simulink model "ssc_battery_management_R2020a"  (R2020a)
settings: Solver=daessc  StartTime=0.0  StopTime=2000  FixedStep=0.1  MinStep=1e-6  RelTol=1e-5  EnableMultiTasking=on
PreLoadFcn:
  | ModelPath = fileparts(get_param(bdroot,'FileName'));
  | addpath(ModelPath);
  | 
  | ssc_battery_management_R2012b_ini
values from neighbouring files (symbols this model uses):
  AltData100AMaxCurrent =     [AlternatorTableData.mat]
  AltData100AVoltage =     [AlternatorTableData.mat]
  AltData80AMaxCurrent =     [AlternatorTableData.mat]
  AltData80AVoltage =     [AlternatorTableData.mat]
  Kt = [0.80,1.10,1.20,1.12;]    [ssc_lead_acid_battery_50Ah_ini.m]    (also in ssc_lead_acid_battery_80Ah_ini.m)
  Kt_Temps = [25 40 60 75]    [ssc_lead_acid_battery_50Ah_ini.m]    (also in ssc_lead_acid_battery_80Ah_ini.m)
  theta_f = -40    [ssc_lead_acid_battery_50Ah_ini.m]    (also in ssc_lead_acid_battery_80Ah_ini.m)
  theta_init = 25    [ssc_lead_acid_battery_50Ah_ini.m]    (also in ssc_lead_acid_battery_80Ah_ini.m)
undefined symbols (not defined in the file or in its folder): beta, center, DiscIntNeverNeededParam, exponent, polyTerms, sigbuilder_block, WendlandNumTerms, width
libraries: fl_lib x130, LeadAcidBattery_lib x36, nesl_utility x28, simulink x6
(part 1 of 4)
settings Model: Creator=smiller  LastModifiedBy=rjack
settings SolverCC: MaxConsecutiveMinStep=10  ZeroCrossAlgorithm=Adaptive  SolverResetMethod=Robust
settings DataIOCC: LimitDataPoints=on  SaveFormat=Array  SignalLoggingSaveFormat=ModelDataLogs  SignalLoggingName=sigsOut
settings OptimizationCC: ExpressionDepthLimit=2147483647  InitFltsAndDblsToZero=on  LifeSpan=inf
settings DebuggingCC: AlgebraicLoopMsg=none  SaveWithParameterizedLinksMsg=none  SignalResolutionControl=TryResolveAllWithWarning  IgnoredZcDiagnostic=none  MultiTaskDSMMsg=warning  MultiTaskCondExecSysMsg=none  StateNameClashWarn=warning  SFUnexpectedBacktrackingDiag=warning  SFNoUnconditionalDefaultTransitionDiag=warning  SFExecutionAtInitializationDiag=none  ArithmeticOperatorsInVariantConditions=warning
settings HardwareCC: ProdBitPerPointer=32  ProdBitPerSizeT=32  ProdBitPerPtrDiffT=32  ProdLargestAtomicFloat=None  ProdIntDivRoundTo=Undefined  ProdEndianess=Unspecified  ProdWordSize=32  ProdHWDeviceType=32-bit Generic  TargetBitPerPointer=64  TargetBitPerSizeT=64  TargetBitPerPtrDiffT=64  TargetLongLongMode=on  TargetIntDivRoundTo=Zero  TargetEndianess=LittleEndian  TargetWordSize=64  TargetHWDeviceType=MATLAB Host  ProdEqTarget=off
settings ModelReferenceCC: PropagateSignalLabelsOutOfModel=off
settings SFSimCC: SimUseLocalCustomCode=off  SimParseCustomCode=off  CustomCodeUndefinedFunction=UseInterfaceOnly
settings RTWCC: RTWUseLocalCustomCode=off
settings CodeAppCC: StateflowObjectComments=on
settings GRTTargetCC: TargetFcnLib=ansi_tfl_tmw.mat  TargetLangStandard=C89/C90 (ANSI)  CombineOutputUpdateFcns=off  GRTInterface=on
settings ConfigComp: CovMetricSettings=dw  CovHtmlReporting=on  CovSaveCumulativeToWorkspaceVar=on  CovSaveSingleToWorkspaceVar=on  CovExternalEMLEnable=off
settings SimscapeCC: SimscapeNormalizeSystem=off

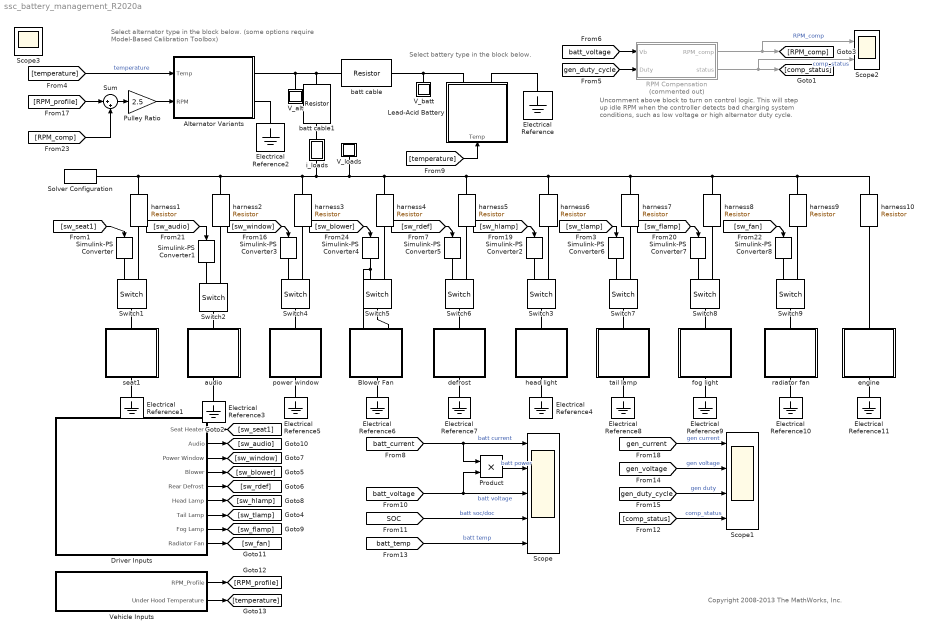
== system ssc_battery_management_R2020a ==
  note: Uncomment above block to turn on control logic.
      | This will step up idle RPM when the controller
      | detects bad charging system conditions, such
      | as low voltage or high alternator duty cycle.
  note: Copyright 2008-2013 The MathWorks, Inc.
  note: Select alternator type in the block below.
      | (some options require Model-Based Calibration Toolbox)
  note: Select battery type in the block below.
  Alternator Variants : Subsystem  Variant=on  mask(Alternator Variants){alt_type=80A (Lookup Tables), i_init=30}
      mask prompts: alt_type "Alternator Size and Type"; i_init "Initial Current (Amperes)"
      mask help:
      | Select from different alternator sizes and types. The Alternator Type selection will update the variable AlternatorSelection in the base workspace, which triggers the variant selection. Look under the mask to view the different alternator models. The initial current sets the initial condition of the alternator's output.
      |
      | The MBC alternator selections require Model-Based Calibration Toolbox to be installed.
      mask init:
      | assignin('base','AlternatorSelection',alt_type)
      mask TypeOptions alt_type: 80A (Lookup Tables) | 100A (Lookup Tables) | 80A (MBC Toolbox - high fidelity) | 100A (MBC Toolbox - high fidelity)
  Blower Fan : Subsystem  mask{steps=[1 2 3 4], current=[2.6 5.8 10 15.1; 2.5 6.4 10.9 16.4; 3.2 7.2 12.3 18.5], voltage=[11 12 13.5]}
      mask Display:
      | plot([45.5890141893179;79.6036154497415;90.9418158698828;113.618216710165;136.294617550448;158.97101839073;181.647419231013;204.323820071295;227.000220911577;249.67662175186;261.014822172001;295.029423432425], [85.2727156598121;85.2727156598121;107.949116500095;62.5963148195297;107.949116500095;62.5963148195297;107.949116500095;62.5963148195297;107.949116500095;62.5963148195297;85.2727156598121;85.2727156598121])
      | plot([0.236212508752999;45.5890141893179;45.5890141893179], [56.927214609459;56.927214609459;85.2727156598121])
      | plot([295.029423432425;295.029423432425;340.38222511299], [85.2727156598121;113.618216710165;113.618216710165])
      | plot([0.236212508752999;45.5890141893179;102.280016290024;124.956417130306;232.669321121648], [170.309218810871;170.309218810871;170.309218810871;141.963717760518;20.0780632440001])
      | plot([209.992920281366;232.669321121648;232.669321121648], [20.0780632440001;20.0780632440001;42.7544640842825])
      | patch([5.6843418860808e-14;340.618437621743;340.618437621743;0;5.6843418860808e-14;0.472425017505941;0.472425017505941;340.146012604237;340.146012604237;0.472425017505941;5.6843418860808e-14], [227.23643342033;227.23643342033;0;0;227.23643342033;226.764008402824;0.472425017505884;0.472425017505884;226.764008402824;226.764008402824;227.23643342033], [1;1;1])
      | ;
      | color('red');
      | port_label('LConn', 1,'Step')
      | port_label('LConn', 2,'+')
      | port_label('RConn', 1,'-')
  Driver Inputs : Subsystem  Tag=STV Subsys  LoadFcn=sigbuilder_block('load');  StartFcn=sigbuilder_block('start');  StopFcn=sigbuilder_block('stop');  ClipboardFcn=sigbuilder_block('clipboard');  mask(Sigbuilder block){tuvar=[0:10]}
      mask help: Sigbuilder GUI
      mask init:
      | if ~strcmp(get_param(bdroot,'SimulationStatus'),'stopped') tuvar = sigbuilder_block('maskInit'); end
      settings: CopyFcn=sigbuilder_block('copy');  DeleteFcn=sigbuilder_block('delete');  ModelCloseFcn=sigbuilder_block('modelClose');  PreSaveFcn=sigbuilder_block('preSave');  PauseFcn=sigbuilder_block('pause')  ContinueFcn=sigbuilder_block('continue')  NameChangeFcn=sigbuilder_block('namechange');  OpenFcn=sigbuilder_block('open',[652.8 249 792.6 639 ]);  CloseFcn=sigbuilder_block('close');
      mask Display: plot(0, 0, 100, 100,[2, 2, 32, 32, 2], [68, 8, 8, 68, 68],[32, 2], [38, 38], [32, 19, 2],[53, 60, 44], [32, 17, 17, 2],[16, 16, 31, 31]);txt = getActiveGroup(gcbh);text(2, 100, txt,'verticalAlignment', 'top');
  Electrical Reference{,1..11} (12 alike) : fl_lib/Electrical/Electrical Elements/Electrical Reference
  Lead-Acid Battery : Subsystem  InitFcn=ssc_lead_acid_battery_50Ah_ini  mask(Lead-Acid Battery){battery_type=50}
      mask prompts: battery_type "Capacity (Ampere-hours)"
      mask help: Select from different battery sizes. The selection will run the corresponding parameter initialization file for the battery capacity selected.
      mask init:
      | switch battery_type
      |     case 1 %50 Ah
      |         ssc_lead_acid_battery_50Ah_ini;
      |     case 2 %80 Ah
      |         ssc_lead_acid_battery_80Ah_ini;
      | end
      mask TypeOptions battery_type: 50 | 80
      mask Display:
      | port_label('RConn',1,'+')
      | port_label('RConn',2,'-')
      | port_label('input',1,'Temp')
      | disp([battery_type ' Ah'])
  Product : Product  RndMeth=Zero
  Pulley Ratio : Gain  Gain=2.5
  RPM Compensation : Subsystem  Commented=on
  Scope : Scope  NumInputPorts=5
  Scope1 : Scope  NumInputPorts=4
  Scope2 : Scope  NumInputPorts=2
  Simulink-PS Converter{,1..8} (9 alike) : nesl_utility/Simulink-PS Converter  PhysicalDomain=network_engine_domain  SubClassName=ps_input  LeftPortType=input  RightPortType=output  PseudoPeriodic=off  Frequencies=[]  NoiseDistribution=none  NoiseParameters=[]  Unit=1  AffineConversion=off  FilteringAndDerivatives=zero  SimscapeFilterOrder=1  InputFilterTimeConstant=.001  UdotUserProvided=0
  Solver Configuration : nesl_utility/Solver Configuration  PhysicalDomain=network_engine_domain  SubClassName=solver  LeftPortType=input  RightPortType=generic  Tones=[]  Harmonics=[]  SimulateNoise=off  Profile=off  UseLocalSampling=off  EnableSwitchedLinearOptims=on  FrequencyDomain=off  UseCCode=off  RelTol=0.001  AbsTol=1e-06  MinStep=1e-09  ToWorkspace=off  RevertToSquareIcSolve=off  NumHomotopyIterations=100  PhasorMode=off  PhasorModeNumHarmonics=1  DoDC=off  ResidualTolerance=1e-6  UseLocalSolver=off  LocalSolverChoice=NE_BACKWARD_EULER_ADVANCER  LocalSolverSampleTime=.001  DoFixedCost=off  MaxNonlinIter=12  MaxModeIter=2  LinearAlgebra=Sparse  EquationFormulation=NE_TIME_EF  DelaysMemoryBudget=1024  AutomaticFiltering=on  FilteringTimeConstant=0.001  PartitionStorageMethod=AS_NEEDED  PartitionMemoryBudget=1024  PartitionMethod=FAST
  Sum : Sum  Inputs=|++
  Switch{1..9} (9 alike) : fl_lib/Electrical/Electrical Elements/Switch  R_closed=0.01 Ohm  G_open=1e-08 1/Ohm  Threshold=0  i_specify=off  i_priority=None  i=0 A  i_nominal_specify=off  i_nominal_unit=A  i_nominal_value=1  v_specify=off  v_priority=None  v=0 V  v_nominal_specify=off  v_nominal_unit=V  v_nominal_value=1
  V_alt : Subsystem  InitFcn=|
      | unit=get_param([gcb '/PS-S'],'Unit');
      | set_param(gcb, 'AttributesFormatString', strcat('[', unit,']'));
      mask help: Simscape Probe
      settings: AttributesFormatString=[V]
      settings: CopyFcn=|
      | set_param(gcb,'LinkStatus','inactive')
      | set_param(gcb,'LinkStatus','none')
      | set_param([gcb '/Goto'],'GotoTag', [get(gcbh,'name')])
      | 
      | set_param([gcb '/From'],'GotoTag', [get(gcbh,'name')])
      settings: NameChangeFcn=|
      | set_param([gcb '/Goto'],'GotoTag', [get(gcbh,'name')])
      | 
      | set_param([gcb '/From'],'GotoTag', [get(gcbh,'name')])
      settings: OpenFcn=|
      | open_system([gcb '/voltage']);
      | close_system(gcb);                    hh=findobj(allchild(0),'name','voltage');
      | ha=findobj(hh(1),'type','axes');
      | set(get(ha,'title'),'string',get(gcbh,'name'));
      | clear hh ha;
      mask Display: port_label('LConn', 1,'V');
  V_batt : Subsystem  InitFcn=|
      | unit=get_param([gcb '/PS-S'],'Unit');
      | set_param(gcb, 'AttributesFormatString', strcat('[', unit,']'));
      mask help: Simscape Probe
      settings: AttributesFormatString=[V]
      settings: CopyFcn=|
      | set_param(gcb,'LinkStatus','inactive')
      | set_param(gcb,'LinkStatus','none')
      | set_param([gcb '/Goto'],'GotoTag', [get(gcbh,'name')])
      | 
      | set_param([gcb '/From'],'GotoTag', [get(gcbh,'name')])
      settings: NameChangeFcn=|
      | set_param([gcb '/Goto'],'GotoTag', [get(gcbh,'name')])
      | 
      | set_param([gcb '/From'],'GotoTag', [get(gcbh,'name')])
      settings: OpenFcn=|
      | open_system([gcb '/voltage']);
      | close_system(gcb);                    hh=findobj(allchild(0),'name','voltage');
      | ha=findobj(hh(1),'type','axes');
      | set(get(ha,'title'),'string',get(gcbh,'name'));
      | clear hh ha;
      mask Display: port_label('LConn', 1,'V');
  V_loads : Subsystem  InitFcn=|
      | unit=get_param([gcb '/PS-S'],'Unit');
      | set_param(gcb, 'AttributesFormatString', strcat('[', unit,']'));
      mask help: Simscape Probe
      settings: AttributesFormatString=[V]
      settings: CopyFcn=|
      | set_param(gcb,'LinkStatus','inactive')
      | set_param(gcb,'LinkStatus','none')
      | set_param([gcb '/Goto'],'GotoTag', [get(gcbh,'name')])
      | 
      | set_param([gcb '/From'],'GotoTag', [get(gcbh,'name')])
      settings: NameChangeFcn=|
      | set_param([gcb '/Goto'],'GotoTag', [get(gcbh,'name')])
      | 
      | set_param([gcb '/From'],'GotoTag', [get(gcbh,'name')])
      settings: OpenFcn=|
      | open_system([gcb '/voltage']);
      | close_system(gcb);                    hh=findobj(allchild(0),'name','voltage');
      | ha=findobj(hh(1),'type','axes');
      | set(get(ha,'title'),'string',get(gcbh,'name'));
      | clear hh ha;
      mask Display: port_label('LConn', 1,'V');
  Vehicle Inputs : Subsystem  Tag=STV Subsys  LoadFcn=sigbuilder_block('load');  StartFcn=sigbuilder_block('start');  StopFcn=sigbuilder_block('stop');  ClipboardFcn=sigbuilder_block('clipboard');  mask(Sigbuilder block){tuvar=[0:10]}
      mask help: Sigbuilder GUI
      mask init:
      | if ~strcmp(get_param(bdroot(gcbh),'SimulationStatus'),'stopped') tuvar = sigbuilder_block('maskInit'); end
      settings: CopyFcn=sigbuilder_block('copy');  DeleteFcn=sigbuilder_block('delete');  ModelCloseFcn=sigbuilder_block('modelClose');  PreSaveFcn=sigbuilder_block('preSave');  PauseFcn=sigbuilder_block('pause')  ContinueFcn=sigbuilder_block('continue')  NameChangeFcn=sigbuilder_block('namechange');  OpenFcn=sigbuilder_block('open',[910.5 430.5 511.5 350.25 ]);  CloseFcn=sigbuilder_block('close');
      mask Display: plot(0, 0, 100, 100,[2, 2, 32, 32, 2], [68, 8, 8, 68, 68],[32, 2], [38, 38], [32, 19, 2],[53, 60, 44], [32, 17, 17, 2],[16, 16, 31, 31]);txt = getActiveGroup(gcbh);text(2, 100, txt,'verticalAlignment', 'top');
  audio : Subsystem  mask{current=[7.64 8.33 9.38], voltage=[11 12 13.5]}
      mask Display:
      | plot([0.236212508752942;34.2508137691766;45.5890141893178;68.2654150296003;90.9418158698827;113.618216710165;136.294617550448;158.97101839073;181.647419231012;204.323820071295;215.662020491436;249.67662175186], [85.2727156598121;85.2727156598121;107.949116500095;62.5963148195297;107.949116500095;62.5963148195297;107.949116500095;62.5963148195297;107.949116500095;62.5963148195297;85.2727156598121;85.2727156598121])
      | plot([50;200], [155;20])
      | plot([170;200;200], [25;20;45])
      | patch([0;249.912834260613;249.912834260613;0;0;0.472425017505884;0.472425017505884;249.440409243107;249.440409243107;0.472425017505884;0], [170.545431319624;170.545431319624;0;0;170.545431319624;170.073006302118;0.472425017505884;0.472425017505884;170.073006302118;170.073006302118;170.545431319624], [1;1;1])
      | ;
      | color('red');
      | port_label('LConn', 1,'+')
      | port_label('RConn', 1,'-')
  batt cable1 : fl_lib/Electrical/Electrical Elements/Resistor  R=0.003 Ohm  i_specify=off  i_priority=None  i=0 A  i_nominal_specify=off  i_nominal_unit=A  i_nominal_value=1  v_specify=off  v_priority=None  v=0 V  v_nominal_specify=off  v_nominal_unit=V  v_nominal_value=1
  batt cable : fl_lib/Electrical/Electrical Elements/Resistor  R=0.03 Ohm  i_specify=off  i_priority=None  i=0 A  i_nominal_specify=off  i_nominal_unit=A  i_nominal_value=1  v_specify=off  v_priority=None  v=0 V  v_nominal_specify=off  v_nominal_unit=V  v_nominal_value=1
  defrost : Subsystem  mask{current=[22.92 25 28.13], voltage=[11 12 13.5]}
      mask Display:
      | plot([0.236212508752942;34.2508137691766;45.5890141893178;68.2654150296003;90.9418158698827;113.618216710165;136.294617550448;158.97101839073;181.647419231012;204.323820071295;215.662020491436;249.67662175186], [85.2727156598121;85.2727156598121;107.949116500095;62.5963148195297;107.949116500095;62.5963148195297;107.949116500095;62.5963148195297;107.949116500095;62.5963148195297;85.2727156598121;85.2727156598121])
      | plot([50;200], [155;20])
      | plot([170;200;200], [25;20;45])
      | patch([0;249.912834260613;249.912834260613;0;0;0.472425017505884;0.472425017505884;249.440409243107;249.440409243107;0.472425017505884;0], [170.545431319624;170.545431319624;0;0;170.545431319624;170.073006302118;0.472425017505884;0.472425017505884;170.073006302118;170.073006302118;170.545431319624], [1;1;1])
      | ;
      | color('red');
      | port_label('LConn', 1,'+')
      | port_label('RConn', 1,'-')
  engine : Subsystem  mask{current=[11.8 12.9 14.5], voltage=[11 12 13.5]}
      mask Display:
      | plot([0.236212508752942;34.2508137691766;45.5890141893178;68.2654150296003;90.9418158698827;113.618216710165;136.294617550448;158.97101839073;181.647419231012;204.323820071295;215.662020491436;249.67662175186], [85.2727156598121;85.2727156598121;107.949116500095;62.5963148195297;107.949116500095;62.5963148195297;107.949116500095;62.5963148195297;107.949116500095;62.5963148195297;85.2727156598121;85.2727156598121])
      | plot([50;200], [155;20])
      | plot([170;200;200], [25;20;45])
      | patch([0;249.912834260613;249.912834260613;0;0;0.472425017505884;0.472425017505884;249.440409243107;249.440409243107;0.472425017505884;0], [170.545431319624;170.545431319624;0;0;170.545431319624;170.073006302118;0.472425017505884;0.472425017505884;170.073006302118;170.073006302118;170.545431319624], [1;1;1])
      | ;
      | color('red');
      | port_label('LConn', 1,'+')
      | port_label('RConn', 1,'-')
  fog light : Subsystem  mask{current=[7.64 8.33 9.38], voltage=[11 12 13.5]}
      mask Display:
      | plot([0.236212508752942;34.2508137691766;45.5890141893178;68.2654150296003;90.9418158698827;113.618216710165;136.294617550448;158.97101839073;181.647419231012;204.323820071295;215.662020491436;249.67662175186], [85.2727156598121;85.2727156598121;107.949116500095;62.5963148195297;107.949116500095;62.5963148195297;107.949116500095;62.5963148195297;107.949116500095;62.5963148195297;85.2727156598121;85.2727156598121])
      | plot([50;200], [155;20])
      | plot([170;200;200], [25;20;45])
      | patch([0;249.912834260613;249.912834260613;0;0;0.472425017505884;0.472425017505884;249.440409243107;249.440409243107;0.472425017505884;0], [170.545431319624;170.545431319624;0;0;170.545431319624;170.073006302118;0.472425017505884;0.472425017505884;170.073006302118;170.073006302118;170.545431319624], [1;1;1])
      | ;
      | color('red');
      | port_label('LConn', 1,'+')
      | port_label('RConn', 1,'-')
  harness{1..8,10} (9 alike) : fl_lib/Electrical/Electrical Elements/Resistor  R=0.05 Ohm  i_specify=off  i_priority=None  i=0 A  i_nominal_specify=off  i_nominal_unit=A  i_nominal_value=1  v_specify=off  v_priority=None  v=0 V  v_nominal_specify=off  v_nominal_unit=V  v_nominal_value=1
  harness9 : fl_lib/Electrical/Electrical Elements/Resistor  R=0.01 Ohm  i_specify=off  i_priority=None  i=0 A  i_nominal_specify=off  i_nominal_unit=A  i_nominal_value=1  v_specify=off  v_priority=None  v=0 V  v_nominal_specify=off  v_nominal_unit=V  v_nominal_value=1
  head light : Subsystem  mask{current=[7.64 8.33 9.38], voltage=[11 12 13.5]}
      mask Display:
      | plot([0.236212508752942;34.2508137691766;45.5890141893178;68.2654150296003;90.9418158698827;113.618216710165;136.294617550448;158.97101839073;181.647419231012;204.323820071295;215.662020491436;249.67662175186], [85.2727156598121;85.2727156598121;107.949116500095;62.5963148195297;107.949116500095;62.5963148195297;107.949116500095;62.5963148195297;107.949116500095;62.5963148195297;85.2727156598121;85.2727156598121])
      | plot([50;200], [155;20])
      | plot([170;200;200], [25;20;45])
      | patch([0;249.912834260613;249.912834260613;0;0;0.472425017505884;0.472425017505884;249.440409243107;249.440409243107;0.472425017505884;0], [170.545431319624;170.545431319624;0;0;170.545431319624;170.073006302118;0.472425017505884;0.472425017505884;170.073006302118;170.073006302118;170.545431319624], [1;1;1])
      | ;
      | color('red');
      | port_label('LConn', 1,'+')
      | port_label('RConn', 1,'-')
  i_loads : Subsystem  InitFcn=|
      | unit=get_param([gcb '/PS-S'],'Unit');
      | set_param(gcb, 'AttributesFormatString', strcat('[', unit,']'));
      mask help: Simscape Probe
      settings: AttributesFormatString=[A]
      settings: CopyFcn=|
      | set_param(gcb,'LinkStatus','inactive')
      | set_param(gcb,'LinkStatus','none')
      | set_param([gcb '/Goto'],'GotoTag', [get(gcbh,'name')])
      | 
      | set_param([gcb '/From'],'GotoTag', [get(gcbh,'name')])
      settings: NameChangeFcn=|
      | set_param([gcb '/Goto'],'GotoTag', [get(gcbh,'name')])
      | 
      | set_param([gcb '/From'],'GotoTag', [get(gcbh,'name')])
      settings: OpenFcn=|
      | open_system([gcb '/current']);
      | close_system(gcb);                    hh=findobj(allchild(0),'name','current');
      | ha=findobj(hh(1),'type','axes');
      | set(get(ha,'title'),'string',get(gcbh,'name'));
      | clear hh ha;
      mask Display:
      | patch([0.5 1 0.5], [0.25 .5 0.75],[0 0 0])
      | plot([0,0.5],[0.5,0.5]);
  power window : Subsystem  mask{current=[7.64 8.33 9.38], voltage=[11 12 13.5]}
      mask Display:
      | plot([0.236212508752942;34.2508137691766;45.5890141893178;68.2654150296003;90.9418158698827;113.618216710165;136.294617550448;158.97101839073;181.647419231012;204.323820071295;215.662020491436;249.67662175186], [85.2727156598121;85.2727156598121;107.949116500095;62.5963148195297;107.949116500095;62.5963148195297;107.949116500095;62.5963148195297;107.949116500095;62.5963148195297;85.2727156598121;85.2727156598121])
      | plot([50;200], [155;20])
      | plot([170;200;200], [25;20;45])
      | patch([0;249.912834260613;249.912834260613;0;0;0.472425017505884;0.472425017505884;249.440409243107;249.440409243107;0.472425017505884;0], [170.545431319624;170.545431319624;0;0;170.545431319624;170.073006302118;0.472425017505884;0.472425017505884;170.073006302118;170.073006302118;170.545431319624], [1;1;1])
      | ;
      | color('red');
      | port_label('LConn', 1,'+')
      | port_label('RConn', 1,'-')
  radiator fan : Subsystem  mask{current=[15.28 16.67 18.75], voltage=[11 12 13.5]}
      mask Display:
      | plot([0.236212508752942;34.2508137691766;45.5890141893178;68.2654150296003;90.9418158698827;113.618216710165;136.294617550448;158.97101839073;181.647419231012;204.323820071295;215.662020491436;249.67662175186], [85.2727156598121;85.2727156598121;107.949116500095;62.5963148195297;107.949116500095;62.5963148195297;107.949116500095;62.5963148195297;107.949116500095;62.5963148195297;85.2727156598121;85.2727156598121])
      | plot([50;200], [155;20])
      | plot([170;200;200], [25;20;45])
      | patch([0;249.912834260613;249.912834260613;0;0;0.472425017505884;0.472425017505884;249.440409243107;249.440409243107;0.472425017505884;0], [170.545431319624;170.545431319624;0;0;170.545431319624;170.073006302118;0.472425017505884;0.472425017505884;170.073006302118;170.073006302118;170.545431319624], [1;1;1])
      | ;
      | color('red');
      | port_label('LConn', 1,'+')
      | port_label('RConn', 1,'-')
  seat1 : Subsystem  mask{current=[11.16 12.5 14.06], voltage=[11 12 13.5]}
      mask Display:
      | plot([0.236212508752942;34.2508137691766;45.5890141893178;68.2654150296003;90.9418158698827;113.618216710165;136.294617550448;158.97101839073;181.647419231012;204.323820071295;215.662020491436;249.67662175186], [85.2727156598121;85.2727156598121;107.949116500095;62.5963148195297;107.949116500095;62.5963148195297;107.949116500095;62.5963148195297;107.949116500095;62.5963148195297;85.2727156598121;85.2727156598121])
      | plot([50;200], [155;20])
      | plot([170;200;200], [25;20;45])
      | patch([0;249.912834260613;249.912834260613;0;0;0.472425017505884;0.472425017505884;249.440409243107;249.440409243107;0.472425017505884;0], [170.545431319624;170.545431319624;0;0;170.545431319624;170.073006302118;0.472425017505884;0.472425017505884;170.073006302118;170.073006302118;170.545431319624], [1;1;1])
      | ;
      | color('red');
      | port_label('LConn', 1,'+')
      | port_label('RConn', 1,'-')
  tail lamp : Subsystem  mask{current=[4.7 4.9 5.15], voltage=[11 12 13.5]}
      mask Display:
      | plot([0.236212508752942;34.2508137691766;45.5890141893178;68.2654150296003;90.9418158698827;113.618216710165;136.294617550448;158.97101839073;181.647419231012;204.323820071295;215.662020491436;249.67662175186], [85.2727156598121;85.2727156598121;107.949116500095;62.5963148195297;107.949116500095;62.5963148195297;107.949116500095;62.5963148195297;107.949116500095;62.5963148195297;85.2727156598121;85.2727156598121])
      | plot([50;200], [155;20])
      | plot([170;200;200], [25;20;45])
      | patch([0;249.912834260613;249.912834260613;0;0;0.472425017505884;0.472425017505884;249.440409243107;249.440409243107;0.472425017505884;0], [170.545431319624;170.545431319624;0;0;170.545431319624;170.073006302118;0.472425017505884;0.472425017505884;170.073006302118;170.073006302118;170.545431319624], [1;1;1])
      | ;
      | color('red');
      | port_label('LConn', 1,'+')
      | port_label('RConn', 1,'-')
  Scope3 : Scope
  wires:
  [batt_current] -> Scope/1, Product/1  "batt current"
  [batt_voltage] -> Scope/3, Product/2  "batt voltage"
  [batt_temp] -> Scope/5  "batt temp"
  Driver Inputs/5(Rear Defrost) -> [sw_rdef]
  Driver Inputs/3(Power Window) -> [sw_window]
  Driver Inputs/6(Head Lamp) -> [sw_hlamp]
  Driver Inputs/8(Fog Lamp) -> [sw_flamp]
  Driver Inputs/2(Audio) -> [sw_audio]
  Driver Inputs/1(Seat Heater) -> [sw_seat1]
  Driver Inputs/9(Radiator Fan) -> [sw_fan]
  [sw_seat1] -> Simulink-PS Converter/1
  [SOC] -> Scope/4  "batt soc/doc"
  Product/1 -> Scope/2  "batt power"
  Vehicle Inputs/1(RPM_Profile) -> [RPM_profile]
  Vehicle Inputs/2(Under Hood Temperature) -> [temperature]
  [temperature] -> Lead-Acid Battery/1(Temp)
  [temperature] -> Alternator Variants/1(Temp)  "temperature"
  Pulley Ratio/1 -> Alternator Variants/2(RPM)
  [sw_audio] -> Simulink-PS Converter1/1
  [sw_window] -> Simulink-PS Converter3/1
  [sw_blower] -> Simulink-PS Converter4/1
  [sw_rdef] -> Simulink-PS Converter5/1
  [sw_tlamp] -> Simulink-PS Converter6/1
  [sw_flamp] -> Simulink-PS Converter7/1
  [sw_fan] -> Simulink-PS Converter8/1
  [sw_hlamp] -> Simulink-PS Converter2/1
  Driver Inputs/7(Tail Lamp) -> [sw_tlamp]
  Driver Inputs/4(Blower) -> [sw_blower]
  [gen_duty_cycle] -> RPM Compensation/2(Duty)
  [batt_voltage] -> RPM Compensation/1(Vb)
  RPM Compensation/2(status) -> [comp_status], Scope2/2  "comp_status"
  RPM Compensation/1(RPM_comp) -> [RPM_comp], Scope2/1  "RPM_comp"
  [RPM_profile] -> Sum/1
  [RPM_comp] -> Sum/2
  Sum/1 -> Pulley Ratio/1
  [gen_current] -> Scope1/1  "gen current"
  [gen_voltage] -> Scope1/2  "gen voltage"
  [gen_duty_cycle] -> Scope1/3  "gen duty"
  [comp_status] -> Scope1/4  "comp_status"
  connections:
  Lead-Acid Battery/RConn2 -- Electrical Reference/LConn1
  Lead-Acid Battery/RConn1 -- batt cable/LConn1 -- V_batt/LConn1
  i_loads/RConn1 -- V_loads/LConn1 -- harness10/LConn1 -- harness9/LConn1 -- harness8/LConn1 -- harness7/LConn1 -- harness6/LConn1 -- harness5/LConn1 -- harness4/LConn1 -- harness3/LConn1 -- harness1/LConn1 -- Solver Configuration/RConn1 -- harness2/LConn1
  Electrical Reference1/LConn1 -- seat1/RConn1
  Simulink-PS Converter/RConn1 -- Switch1/RConn1
  harness1/RConn1 -- Switch1/RConn2
  seat1/LConn1 -- Switch1/LConn1
  engine/LConn1 -- harness10/RConn1
  Electrical Reference11/LConn1 -- engine/RConn1
  batt cable/RConn1 -- Alternator Variants/RConn1 -- V_alt/LConn1 -- batt cable1/LConn1
  Alternator Variants/RConn2 -- Electrical Reference2/LConn1
  Switch2/LConn1 -- audio/LConn1
  Simulink-PS Converter1/RConn1 -- Switch2/RConn1
  Electrical Reference3/LConn1 -- audio/RConn1
  Electrical Reference4/LConn1 -- head light/RConn1
  Simulink-PS Converter2/RConn1 -- Switch3/RConn1
  Switch3/LConn1 -- head light/LConn1
  Electrical Reference5/LConn1 -- power window/RConn1
  Switch4/LConn1 -- power window/LConn1
  Simulink-PS Converter3/RConn1 -- Switch4/RConn1
  Switch5/LConn1 -- Blower Fan/LConn2
  Electrical Reference6/LConn1 -- Blower Fan/RConn1
  Simulink-PS Converter5/RConn1 -- Switch6/RConn1
  Switch6/LConn1 -- defrost/LConn1
  Electrical Reference7/LConn1 -- defrost/RConn1
  harness7/RConn1 -- Switch7/RConn2
  Simulink-PS Converter6/RConn1 -- Switch7/RConn1
  Electrical Reference8/LConn1 -- tail lamp/RConn1
  Switch7/LConn1 -- tail lamp/LConn1
  harness8/RConn1 -- Switch8/RConn2
  Electrical Reference9/LConn1 -- fog light/RConn1
  Switch8/LConn1 -- fog light/LConn1
  Simulink-PS Converter7/RConn1 -- Switch8/RConn1
  Simulink-PS Converter8/RConn1 -- Switch9/RConn1
  Switch9/LConn1 -- radiator fan/LConn1
  Electrical Reference10/LConn1 -- radiator fan/RConn1
  harness9/RConn1 -- Switch9/RConn2
  harness5/RConn1 -- Switch6/RConn2
  Switch4/RConn2 -- harness3/RConn1
  harness6/RConn1 -- Switch3/RConn2
  harness2/RConn1 -- Switch2/RConn2
  Blower Fan/LConn1 -- Simulink-PS Converter4/RConn1 -- Switch5/RConn1
  Switch5/RConn2 -- harness4/RConn1
  batt cable1/RConn1 -- i_loads/LConn1

== system ssc_battery_management_R2020a/Alternator Variants ==
  note: 1) Only subsystems can be added as variant choices at this level
      | 2) Blocks cannot be connected at this level as connectivity is
      | automatically determined at simulation, based on the active variant
  note: Alternator Blocks - Lookup Tables
  note: Alternator Blocks - MBC
  Temp : Inport
  RPM : Inport  Port=2
  Alternator_100A_LUT : Subsystem  VariantControl=Alternator_100A_LUT
  Alternator_100A_MBC : Subsystem  VariantControl=Alternator_100A_MBC
  Alternator_80A_LUT : Subsystem  VariantControl=Alternator_80A_LUT
  Alternator_80A_MBC : Subsystem  VariantControl=Alternator_80A_MBC
  + : PMIOPort  Side=Right
  - : PMIOPort  Port=2  Side=Right

== system ssc_battery_management_R2020a/Blower Fan ==
  PS Lookup Table (2D) : fl_lib/Physical Signals/Lookup Tables/PS Lookup Table (2D)  x1=[0 voltage]' V  x2=steps  f="[voltage(1)./current(1,:);  (voltage'*ones(size(steps)))./current] Ohm"  interp_method=simscape.enum.interpolation.linear  extrap_method=simscape.enum.extrapolation.nearest
      settings: SourceProductBaseCode=SS
  Variable Resistor : fl_lib/Electrical/Electrical Elements/Variable Resistor  Rmin=0.01 Ohm  i_specify=off  i_priority=None  i=0 A  i_nominal_specify=off  i_nominal_unit=A  i_nominal_value=1  v_specify=off  v_priority=None  v=0 V  v_nominal_specify=off  v_nominal_unit=V  v_nominal_value=1
  Voltage Sensor : fl_lib/Electrical/Electrical Sensors/Voltage Sensor
  Step : PMIOPort  Tag=PMCPort  Side=Left
  + : PMIOPort  Tag=PMCPort  Port=2  Side=Left
  - : PMIOPort  Tag=PMCPort  Port=3  Side=Right
  connections:
  Step/RConn1 -- PS Lookup Table (2D)/LConn2
  Voltage Sensor/RConn1 -- PS Lookup Table (2D)/LConn1
  +/RConn1 -- Variable Resistor/LConn2 -- Voltage Sensor/LConn1
  -/RConn1 -- Variable Resistor/RConn1 -- Voltage Sensor/RConn2
  Variable Resistor/LConn1 -- PS Lookup Table (2D)/RConn1

== system ssc_battery_management_R2020a/Driver Inputs ==
  Demux : Demux  Tag=STV Demux  Outputs=9
      settings: DisplayOption=none
  FromWs : FromWorkspace  Tag=STV FromWs  VariableName=tuvar  ZeroCross=off
      SigBuilderData=|
      | dataSet(1).timeRange = [0 2000]
      | dataSet(1).name = 'USA'
      | dataSet(2).timeRange = [0 2000]
      | dataSet(2).name = 'Asia'
      | dataSet(3).timeRange = [0 2000]
      | dataSet(3).name = 'Europe'
      | sbobj.Groups(1).Name = 'USA'
      | sbobj.Groups(1).Signals(1).Name = 'Seat Heater'
      | sbobj.Groups(1).Signals(1).XData = [0 60 60 886 886 2000]
      | sbobj.Groups(1).Signals(1).YData = [0 0 1 1 0 0]
      | sbobj.Groups(1).Signals(2).Name = 'Audio'
      | sbobj.Groups(1).Signals(2).XData = [0 116 116 2000]
      | sbobj.Groups(1).Signals(2).YData = [0 0 1 1]
      | sbobj.Groups(1).Signals(3).Name = 'Power Window'
      | sbobj.Groups(1).Signals(3).XData = [0 728 728 740 740 786 786 800 800 2000]
      | sbobj.Groups(1).Signals(3).YData = [0 0 1 1 0 0 1 1 0 0]
      | sbobj.Groups(1).Signals(4).Name = 'Blower'
      | sbobj.Groups(1).Signals(4).XData = [0 50 50 136 136 384 384 820 820 1082 1082 2000]
      | sbobj.Groups(1).Signals(4).YData = [0 0 4 4 3 3 2 2 1 1 2 2]
      | sbobj.Groups(1).Signals(5).Name = 'Rear Defrost'
      | sbobj.Groups(1).Signals(5).XData = [0 20 20 436 436 2000]
      | sbobj.Groups(1).Signals(5).YData = [0 0 1 1 0 0]
      | sbobj.Groups(1).Signals(6).Name = 'Head Lamp'
      | sbobj.Groups(1).Signals(6).XData = [0 200 200 2000]
      | sbobj.Groups(1).Signals(6).YData = [0 0 1 1]
      | sbobj.Groups(1).Signals(7).Name = 'Tail Lamp'
      | sbobj.Groups(1).Signals(7).XData = [0 200 200 2000]
      | sbobj.Groups(1).Signals(7).YData = [0 0 1 1]
      | sbobj.Groups(1).Signals(8).Name = 'Fog Lamp'
      | sbobj.Groups(1).Signals(8).XData = [0 400 400 2000]
      | sbobj.Groups(1).Signals(8).YData = [0 0 1 1]
      | sbobj.Groups(1).Signals(9).Name = 'Radiator Fan'
      | sbobj.Groups(1).Signals(9).XData = [0 814 814 1424 1424 2000]
      | sbobj.Groups(1).Signals(9).YData = [0 0 1 1 0 0]
      | sbobj.Groups(1).TimeRange = [0 2000]
      | sbobj.Groups(2).Name = 'Asia'
      | sbobj.Groups(2).Signals(1).Name = 'Seat Heater'
      | sbobj.Groups(2).Signals(1).XData = [0 60 886 2000]
      | sbobj.Groups(2).Signals(1).YData = [0 0 0 0]
      | sbobj.Groups(2).Signals(2).Name = 'Audio'
      | sbobj.Groups(2).Signals(2).XData = [0 116 116 2000]
      | sbobj.Groups(2).Signals(2).YData = [0 0 1 1]
      | sbobj.Groups(2).Signals(3).Name = 'Power Window'
      | sbobj.Groups(2).Signals(3).XData = [0 312 312 330 330 1762 1762 1774 1774 2000]
      | sbobj.Groups(2).Signals(3).YData = [0 0 1 1 0 0 1 1 0 0]
      | sbobj.Groups(2).Signals(4).Name = 'Blower'
      | sbobj.Groups(2).Signals(4).XData = [0 50 50 136 136 282 282 820 820 1082 1082 2000]
      | sbobj.Groups(2).Signals(4).YData = [0 0 4 4 3 3 -0.1 -0.1 1 1 0 0]
      | sbobj.Groups(2).Signals(5).Name = 'Rear Defrost'
      | sbobj.Groups(2).Signals(5).XData = [0 20 436 2000]
      | sbobj.Groups(2).Signals(5).YData = [0 0 0 0]
      | sbobj.Groups(2).Signals(6).Name = 'Head Lamp'
      | sbobj.Groups(2).Signals(6).XData = [0 200 2000]
      | sbobj.Groups(2).Signals(6).YData = [0 0 0]
      | sbobj.Groups(2).Signals(7).Name = 'Tail Lamp'
      | sbobj.Groups(2).Signals(7).XData = [0 200 2000]
      | sbobj.Groups(2).Signals(7).YData = [0 0 0]
      | sbobj.Groups(2).Signals(8).Name = 'Fog Lamp'
      | sbobj.Groups(2).Signals(8).XData = [0 400 2000]
      | sbobj.Groups(2).Signals(8).YData = [0 0 0]
      | sbobj.Groups(2).Signals(9).Name = 'Radiator Fan'
      | sbobj.Groups(2).Signals(9).XData = [0 810 810 1538 1538 2000]
      | sbobj.Groups(2).Signals(9).YData = [0 0 1 1 0 0]
      | sbobj.Groups(2).TimeRange = [0 2000]
      | sbobj.Groups(3).Name = 'Europe'
      | sbobj.Groups(3).Signals(1).Name = 'Seat Heater'
      | sbobj.Groups(3).Signals(1).XData = [0 164 164 2000]
      | sbobj.Groups(3).Signals(1).YData = [0 0 1 1]
      | sbobj.Groups(3).Signals(2).Name = 'Audio'
      | sbobj.Groups(3).Signals(2).XData = [0 116 116 2000]
      | sbobj.Groups(3).Signals(2).YData = [0 0 1 1]
      | sbobj.Groups(3).Signals(3).Name = 'Power Window'
      | sbobj.Groups(3).Signals(3).XData = [0 728 728 740 740 786 786 800 800 1046 1046 1060 1060 1118 1118 1140 1140 2000]
      | sbobj.Groups(3).Signals(3).YData = [0 0 1 1 0 0 1 1 0 0 1 1 0 0 1 1 0 0]
      | sbobj.Groups(3).Signals(4).Name = 'Blower'
      | sbobj.Groups(3).Signals(4).XData = [0 50 50 136 136 384 384 820 820 1082 1082 2000]
      | sbobj.Groups(3).Signals(4).YData = [0 0 4 4 3 3 2 2 3 3 2 2]
      | sbobj.Groups(3).Signals(5).Name = 'Rear Defrost'
      | sbobj.Groups(3).Signals(5).XData = [0 20 20 496 496 972 972 1660 1660 2000]
      | sbobj.Groups(3).Signals(5).YData = [0 0 1 1 0 0 1 1 0 0]
      | sbobj.Groups(3).Signals(6).Name = 'Head Lamp'
      | sbobj.Groups(3).Signals(6).XData = [0 20 20 2000]
      | sbobj.Groups(3).Signals(6).YData = [0 0 1 1]
      | sbobj.Groups(3).Signals(7).Name = 'Tail Lamp'
      | sbobj.Groups(3).Signals(7).XData = [0 18 720 2000]
      | sbobj.Groups(3).Signals(7).YData = [0 0 0 0]
      | sbobj.Groups(3).Signals(8).Name = 'Fog Lamp'
      | sbobj.Groups(3).Signals(8).XData = [0 400 2000]
      | sbobj.Groups(3).Signals(8).YData = [0 0 0]
      | sbobj.Groups(3).Signals(9).Name = 'Radiator Fan'
      | sbobj.Groups(3).Signals(9).XData = [0 996 996 1198 1198 2000]
      | sbobj.Groups(3).Signals(9).YData = [0 0 1 1 0 0]
      | sbobj.Groups(3).TimeRange = [0 2000]
  Seat Heater : Outport  Tag=STV Outport
  Audio : Outport  Tag=STV Outport  Port=2
  Power Window : Outport  Tag=STV Outport  Port=3
  Blower : Outport  Tag=STV Outport  Port=4
  Rear Defrost : Outport  Tag=STV Outport  Port=5
  Head Lamp : Outport  Tag=STV Outport  Port=6
  Tail Lamp : Outport  Tag=STV Outport  Port=7
  Fog Lamp : Outport  Tag=STV Outport  Port=8
  Radiator Fan : Outport  Tag=STV Outport  Port=9
  wires:
  FromWs/1 -> Demux/1
  Demux/1 -> Seat Heater/1
  Demux/2 -> Audio/1
  Demux/3 -> Power Window/1
  Demux/4 -> Blower/1
  Demux/5 -> Rear Defrost/1
  Demux/6 -> Head Lamp/1
  Demux/7 -> Tail Lamp/1
  Demux/8 -> Fog Lamp/1
  Demux/9 -> Radiator Fan/1

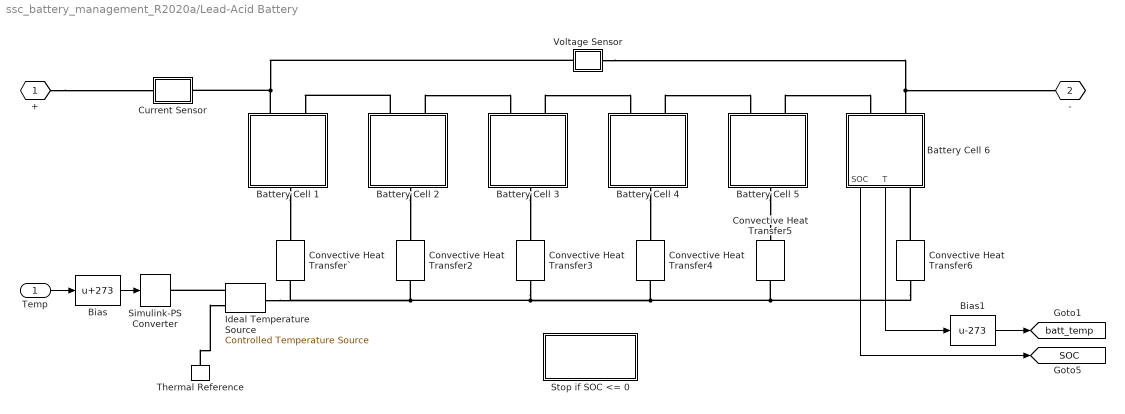
== system ssc_battery_management_R2020a/Lead-Acid Battery ==
  Temp : Inport
  Battery Cell 1 : Subsystem
      mask Display:
      | image('battery.jpg')
      | color('red')
      | port_label('RConn',1,'H')
      | port_label('LConn',1,'+')
      | port_label('LConn',2,'-')
  Battery Cell 2 : Subsystem
      mask Display:
      | image('battery.jpg')
      | color('red')
      | port_label('RConn',1,'H')
      | port_label('LConn',1,'+')
      | port_label('LConn',2,'-')
  Battery Cell 3 : Subsystem
      mask Display:
      | image('battery.jpg')
      | color('red')
      | port_label('RConn',1,'H')
      | port_label('LConn',1,'+')
      | port_label('LConn',2,'-')
  Battery Cell 4 : Subsystem
      mask Display:
      | image('battery.jpg')
      | color('red')
      | port_label('RConn',1,'H')
      | port_label('LConn',1,'+')
      | port_label('LConn',2,'-')
  Battery Cell 5 : Subsystem
      mask Display:
      | image('battery.jpg')
      | color('red')
      | port_label('RConn',1,'H')
      | port_label('LConn',1,'+')
      | port_label('LConn',2,'-')
  Battery Cell 6 : Subsystem
      mask Display:
      | image('battery.jpg')
      | color('red')
      | port_label('RConn',1,'H')
      | port_label('LConn',1,'+')
      | port_label('LConn',2,'-')
      | port_label('output',1,'SOC')
      | port_label('output',2,'T')
  Bias : Bias  Bias=273
  Bias1 : Bias  Bias=-273
  Convective Heat Transfer{2..6} (5 alike) : fl_lib/Thermal/Thermal Elements/Convective Heat Transfer  area=Area m^2  heat_tr_coeff=Rtheta W/(m^2 * K)  T_specify=off  T_priority=None  T=0 K  T_nominal_specify=off  T_nominal_unit=K  T_nominal_value=1  Q_specify=off  Q_priority=None  Q=0 W  Q_nominal_specify=off  Q_nominal_unit=W  Q_nominal_value=1
  Convective Heat Transfer` : fl_lib/Thermal/Thermal Elements/Convective Heat Transfer  area=Area m^2  heat_tr_coeff=Rtheta W/(m^2 * K)  T_specify=off  T_priority=None  T=0 K  T_nominal_specify=off  T_nominal_unit=K  T_nominal_value=1  Q_specify=off  Q_priority=None  Q=0 W  Q_nominal_specify=off  Q_nominal_unit=W  Q_nominal_value=1
  Current Sensor : Subsystem
  Ideal Temperature Source : fl_lib/Thermal/Thermal Sources/Controlled Temperature Source
  Simulink-PS Converter : nesl_utility/Simulink-PS Converter  PhysicalDomain=network_engine_domain  SubClassName=ps_input  LeftPortType=input  RightPortType=output  PseudoPeriodic=off  Frequencies=[]  NoiseDistribution=none  NoiseParameters=[]  Unit=K  AffineConversion=off  FilteringAndDerivatives=zero  SimscapeFilterOrder=1  InputFilterTimeConstant=.001  UdotUserProvided=1
  Stop if SOC <= 0 : Subsystem
  Thermal Reference : fl_lib/Thermal/Thermal Elements/Thermal Reference
  Voltage Sensor : Subsystem
  + : PMIOPort  Tag=PMCPort  Side=Right
  - : PMIOPort  Tag=PMCPort  Port=2  Side=Right
  tag scope: SOC=global, batt_temp=global
  wires:
  Temp/1 -> Bias/1
  Bias/1 -> Simulink-PS Converter/1
  Battery Cell 6/1(SOC) -> [SOC]
  Battery Cell 6/2(T) -> Bias1/1
  Bias1/1 -> [batt_temp]
  connections:
  Voltage Sensor/RConn1 -- -/RConn1 -- Battery Cell 6/LConn2
  +/RConn1 -- Current Sensor/LConn1
  Voltage Sensor/LConn1 -- Battery Cell 1/LConn1 -- Current Sensor/RConn1
  Ideal Temperature Source/RConn1 -- Simulink-PS Converter/RConn1
  Thermal Reference/LConn1 -- Ideal Temperature Source/RConn2
  Battery Cell 1/RConn1 -- Convective Heat Transfer`/RConn1
  Battery Cell 2/RConn1 -- Convective Heat Transfer2/RConn1
  Battery Cell 3/RConn1 -- Convective Heat Transfer3/RConn1
  Battery Cell 4/RConn1 -- Convective Heat Transfer4/RConn1
  Battery Cell 5/RConn1 -- Convective Heat Transfer5/RConn1
  Convective Heat Transfer6/RConn1 -- Battery Cell 6/RConn1
  Convective Heat Transfer6/LConn1 -- Convective Heat Transfer3/LConn1 -- Convective Heat Transfer`/LConn1 -- Ideal Temperature Source/LConn1 -- Convective Heat Transfer2/LConn1 -- Convective Heat Transfer4/LConn1 -- Convective Heat Transfer5/LConn1
  Battery Cell 2/LConn1 -- Battery Cell 1/LConn2
  Battery Cell 2/LConn2 -- Battery Cell 3/LConn1
  Battery Cell 3/LConn2 -- Battery Cell 4/LConn1
  Battery Cell 4/LConn2 -- Battery Cell 5/LConn1
  Battery Cell 5/LConn2 -- Battery Cell 6/LConn1

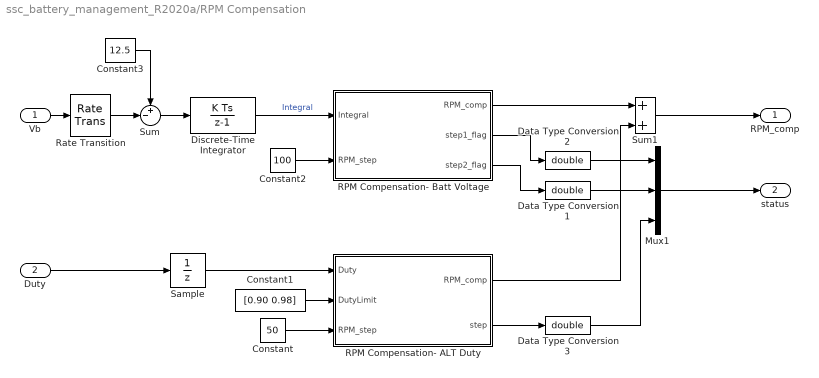
== system ssc_battery_management_R2020a/RPM Compensation ==
  Vb : Inport
  Duty : Inport  Port=2
  Constant : Constant  Value=50
  Constant1 : Constant  Value=[0.90 0.98]
  Constant2 : Constant  Value=100
  Constant3 : Constant  Value=12.5
  Data Type Conversion1 : DataTypeConversion  OutDataTypeStr=double
  Data Type Conversion2 : DataTypeConversion  OutDataTypeStr=double
  Data Type Conversion3 : DataTypeConversion  OutDataTypeStr=double
  Discrete-Time Integrator : DiscreteIntegrator  LimitOutput=on  LowerSaturationLimit=0  ICPrevOutput=DiscIntNeverNeededParam  ICPrevScaledInput=DiscIntNeverNeededParam
  Mux1 : Mux  Inputs=3
  RPM Compensation- ALT Duty : Stateflow chart  TreatAsAtomicUnit=on
  RPM Compensation- Batt Voltage : Stateflow chart  TreatAsAtomicUnit=on
  Rate Transition : RateTransition
  Sample : UnitDelay  HasFrameUpgradeWarning=on
  Sum : Sum  Inputs=+-|  SampleTime=1
  Sum1 : Sum
  RPM_comp : Outport
  status : Outport  Port=2
  wires:
  Constant2/1 -> RPM Compensation- Batt Voltage/2(RPM_step)
  RPM Compensation- Batt Voltage/1(RPM_comp) -> Sum1/1
  Constant1/1 -> RPM Compensation- ALT Duty/2(DutyLimit)
  Constant/1 -> RPM Compensation- ALT Duty/3(RPM_step)
  Discrete-Time Integrator/1 -> RPM Compensation- Batt Voltage/1(Integral)  "Integral"
  Constant3/1 -> Sum/1
  Sum/1 -> Discrete-Time Integrator/1
  RPM Compensation- ALT Duty/1(RPM_comp) -> Sum1/2
  RPM Compensation- ALT Duty/2(step) -> Data Type Conversion3/1
  RPM Compensation- Batt Voltage/2(step1_flag) -> Data Type Conversion2/1
  RPM Compensation- Batt Voltage/3(step2_flag) -> Data Type Conversion1/1
  Vb/1 -> Rate Transition/1
  Sum1/1 -> RPM_comp/1
  Mux1/1 -> status/1
  Duty/1 -> Sample/1
  Data Type Conversion1/1 -> Mux1/2
  Data Type Conversion2/1 -> Mux1/1
  Sample/1 -> RPM Compensation- ALT Duty/1(Duty)
  Data Type Conversion3/1 -> Mux1/3
  Rate Transition/1 -> Sum/2

== system ssc_battery_management_R2020a/V_alt ==
  Electrical Reference : fl_lib/Electrical/Electrical Elements/Electrical Reference
  PS-S : nesl_utility/PS-Simulink Converter  PhysicalDomain=network_engine_domain  SubClassName=ps_output  LeftPortType=input  RightPortType=output  PseudoPeriodic=off  Frequencies=[]  Unit=V  AffineConversion=off
  Terminator : Terminator
  Voltage Sensor : fl_lib/Electrical/Electrical Sensors/Voltage Sensor
  voltage : Scope
  p : PMIOPort  Side=Left
  wires:
  [V_alt] -> Terminator/1
  PS-S/1 -> voltage/1, [V_alt]  "voltage"
  connections:
  p/RConn1 -- Voltage Sensor/LConn1
  PS-S/LConn1 -- Voltage Sensor/RConn1
  Electrical Reference/LConn1 -- Voltage Sensor/RConn2

== system ssc_battery_management_R2020a/V_batt ==
  Electrical Reference : fl_lib/Electrical/Electrical Elements/Electrical Reference
  PS-S : nesl_utility/PS-Simulink Converter  PhysicalDomain=network_engine_domain  SubClassName=ps_output  LeftPortType=input  RightPortType=output  PseudoPeriodic=off  Frequencies=[]  Unit=V  AffineConversion=off
  Terminator : Terminator
  Voltage Sensor : fl_lib/Electrical/Electrical Sensors/Voltage Sensor
  voltage : Scope
  p : PMIOPort  Side=Left
  wires:
  PS-S/1 -> [V_batt], voltage/1  "voltage"
  [V_batt] -> Terminator/1
  connections:
  Electrical Reference/LConn1 -- Voltage Sensor/RConn2
  PS-S/LConn1 -- Voltage Sensor/RConn1
  p/RConn1 -- Voltage Sensor/LConn1

== system ssc_battery_management_R2020a/V_loads ==
  Electrical Reference : fl_lib/Electrical/Electrical Elements/Electrical Reference
  PS-S : nesl_utility/PS-Simulink Converter  PhysicalDomain=network_engine_domain  SubClassName=ps_output  LeftPortType=input  RightPortType=output  PseudoPeriodic=off  Frequencies=[]  Unit=V  AffineConversion=off
  Terminator : Terminator
  Voltage Sensor : fl_lib/Electrical/Electrical Sensors/Voltage Sensor
  voltage : Scope
  p : PMIOPort  Side=Left
  wires:
  [V_loads] -> Terminator/1
  PS-S/1 -> voltage/1, [V_loads]  "voltage"
  connections:
  p/RConn1 -- Voltage Sensor/LConn1
  PS-S/LConn1 -- Voltage Sensor/RConn1
  Electrical Reference/LConn1 -- Voltage Sensor/RConn2

== system ssc_battery_management_R2020a/Vehicle Inputs ==
  Demux : Demux  Tag=STV Demux  Outputs=2
      settings: DisplayOption=none
  FromWs : FromWorkspace  Tag=STV FromWs  VariableName=tuvar
      SigBuilderData=|
      | common.afterFinalStr = 'Extrapolate'
      | common.sampleTime = 0
      | dataSet(1).timeRange = [0 2000]
      | dataSet(1).name = 'ADVISOR'
      | dataSet(2).timeRange = [0 2000]
      | dataSet(2).name = 'Idle'
      | sbobj.Groups(1).Name = 'ADVISOR'
      | sbobj.Groups(1).Signals(1).Name = 'RPM_Profile'
      | sbobj.Groups(1).Signals(1).XData = [0 1 2 3 4 5 6 7 8 9 10 11 ... (2001 elements, 1x2001)]
      | sbobj.Groups(1).Signals(1).YData = [550 550 950.002585738 950.000000073 1838.89007312 1791.36832676 550 550 550 550 550 550 ... (2001 elements, 1x2001)]
      | sbobj.Groups(1).Signals(2).Name = 'Under Hood Temperature'
      | sbobj.Groups(1).Signals(2).XData = [0 500 2000]
      | sbobj.Groups(1).Signals(2).YData = [25 45 45]
      | sbobj.Groups(1).TimeRange = [0 2000]
      | sbobj.Groups(2).Name = 'Idle'
      | sbobj.Groups(2).Signals(1).Name = 'RPM_Profile'
      | sbobj.Groups(2).Signals(1).XData = [0 2000]
      | sbobj.Groups(2).Signals(1).YData = [600 600]
      | sbobj.Groups(2).Signals(2).Name = 'Under Hood Temperature'
      | sbobj.Groups(2).Signals(2).XData = [0 810 2000]
      | sbobj.Groups(2).Signals(2).YData = [25 45 45]
      | sbobj.Groups(2).TimeRange = [0 2000]
  RPM_Profile : Outport  Tag=STV Outport
  Under Hood Temperature : Outport  Tag=STV Outport  Port=2
  wires:
  Demux/1 -> RPM_Profile/1
  FromWs/1 -> Demux/1
  Demux/2 -> Under Hood Temperature/1

== system ssc_battery_management_R2020a/audio ==
  PS Lookup Table (1D) : fl_lib/Physical Signals/Lookup Tables/PS Lookup Table (1D)  x=[0 voltage] V  f=[voltage(1)/current(1) voltage./current] Ohm  interp_method=simscape.enum.interpolation.linear  extrap_method=simscape.enum.extrapolation.nearest
      settings: SourceProductBaseCode=SS
  Variable Resistor : fl_lib/Electrical/Electrical Elements/Variable Resistor  Rmin=0.01 Ohm  i_specify=off  i_priority=None  i=0 A  i_nominal_specify=off  i_nominal_unit=A  i_nominal_value=1  v_specify=off  v_priority=None  v=0 V  v_nominal_specify=off  v_nominal_unit=V  v_nominal_value=1
  Voltage Sensor : fl_lib/Electrical/Electrical Sensors/Voltage Sensor
  + : PMIOPort  Tag=PMCPort  Side=Left
  - : PMIOPort  Tag=PMCPort  Port=2  Side=Right
  connections:
  Voltage Sensor/RConn2 -- Variable Resistor/RConn1 -- -/RConn1
  Voltage Sensor/LConn1 -- Variable Resistor/LConn2 -- +/RConn1
  Voltage Sensor/RConn1 -- PS Lookup Table (1D)/LConn1
  PS Lookup Table (1D)/RConn1 -- Variable Resistor/LConn1

== system ssc_battery_management_R2020a/defrost ==
  PS Lookup Table (1D) : fl_lib/Physical Signals/Lookup Tables/PS Lookup Table (1D)  x=[0 voltage] V  f=[voltage(1)/current(1) voltage./current] Ohm  interp_method=simscape.enum.interpolation.linear  extrap_method=simscape.enum.extrapolation.nearest
      settings: SourceProductBaseCode=SS
  Variable Resistor : fl_lib/Electrical/Electrical Elements/Variable Resistor  Rmin=0.01 Ohm  i_specify=off  i_priority=None  i=0 A  i_nominal_specify=off  i_nominal_unit=A  i_nominal_value=1  v_specify=off  v_priority=None  v=0 V  v_nominal_specify=off  v_nominal_unit=V  v_nominal_value=1
  Voltage Sensor : fl_lib/Electrical/Electrical Sensors/Voltage Sensor
  + : PMIOPort  Tag=PMCPort  Side=Left
  - : PMIOPort  Tag=PMCPort  Port=2  Side=Right
  connections:
  Voltage Sensor/RConn2 -- Variable Resistor/RConn1 -- -/RConn1
  Voltage Sensor/LConn1 -- Variable Resistor/LConn2 -- +/RConn1
  Voltage Sensor/RConn1 -- PS Lookup Table (1D)/LConn1
  PS Lookup Table (1D)/RConn1 -- Variable Resistor/LConn1

== system ssc_battery_management_R2020a/engine ==
  PS Lookup Table (1D) : fl_lib/Physical Signals/Lookup Tables/PS Lookup Table (1D)  x=[0 voltage] V  f=[voltage(1)/current(1) voltage./current] Ohm  interp_method=simscape.enum.interpolation.linear  extrap_method=simscape.enum.extrapolation.nearest
      settings: SourceProductBaseCode=SS
  Variable Resistor : fl_lib/Electrical/Electrical Elements/Variable Resistor  Rmin=0.01 Ohm  i_specify=off  i_priority=None  i=0 A  i_nominal_specify=off  i_nominal_unit=A  i_nominal_value=1  v_specify=off  v_priority=None  v=0 V  v_nominal_specify=off  v_nominal_unit=V  v_nominal_value=1
  Voltage Sensor : fl_lib/Electrical/Electrical Sensors/Voltage Sensor
  + : PMIOPort  Tag=PMCPort  Side=Left
  - : PMIOPort  Tag=PMCPort  Port=2  Side=Right
  connections:
  Variable Resistor/LConn1 -- PS Lookup Table (1D)/RConn1
  Voltage Sensor/RConn2 -- Variable Resistor/RConn1 -- -/RConn1
  Voltage Sensor/LConn1 -- Variable Resistor/LConn2 -- +/RConn1
  Voltage Sensor/RConn1 -- PS Lookup Table (1D)/LConn1

== system ssc_battery_management_R2020a/fog light ==
  PS Lookup Table (1D) : fl_lib/Physical Signals/Lookup Tables/PS Lookup Table (1D)  x=[0 voltage] V  f=[voltage(1)/current(1) voltage./current] Ohm  interp_method=simscape.enum.interpolation.linear  extrap_method=simscape.enum.extrapolation.nearest
      settings: SourceProductBaseCode=SS
  Variable Resistor : fl_lib/Electrical/Electrical Elements/Variable Resistor  Rmin=0.01 Ohm  i_specify=off  i_priority=None  i=0 A  i_nominal_specify=off  i_nominal_unit=A  i_nominal_value=1  v_specify=off  v_priority=None  v=0 V  v_nominal_specify=off  v_nominal_unit=V  v_nominal_value=1
  Voltage Sensor : fl_lib/Electrical/Electrical Sensors/Voltage Sensor
  + : PMIOPort  Tag=PMCPort  Side=Left
  - : PMIOPort  Tag=PMCPort  Port=2  Side=Right
  connections:
  Voltage Sensor/RConn2 -- Variable Resistor/RConn1 -- -/RConn1
  Voltage Sensor/LConn1 -- Variable Resistor/LConn2 -- +/RConn1
  Voltage Sensor/RConn1 -- PS Lookup Table (1D)/LConn1
  PS Lookup Table (1D)/RConn1 -- Variable Resistor/LConn1

== system ssc_battery_management_R2020a/head light ==
  PS Lookup Table (1D) : fl_lib/Physical Signals/Lookup Tables/PS Lookup Table (1D)  x=[0 voltage] V  f=[voltage(1)/current(1) voltage./current] Ohm  interp_method=simscape.enum.interpolation.linear  extrap_method=simscape.enum.extrapolation.nearest
      settings: SourceProductBaseCode=SS
  Variable Resistor : fl_lib/Electrical/Electrical Elements/Variable Resistor  Rmin=0.01 Ohm  i_specify=off  i_priority=None  i=0 A  i_nominal_specify=off  i_nominal_unit=A  i_nominal_value=1  v_specify=off  v_priority=None  v=0 V  v_nominal_specify=off  v_nominal_unit=V  v_nominal_value=1
  Voltage Sensor : fl_lib/Electrical/Electrical Sensors/Voltage Sensor
  + : PMIOPort  Tag=PMCPort  Side=Left
  - : PMIOPort  Tag=PMCPort  Port=2  Side=Right
  connections:
  Voltage Sensor/RConn2 -- Variable Resistor/RConn1 -- -/RConn1
  Voltage Sensor/LConn1 -- Variable Resistor/LConn2 -- +/RConn1
  Voltage Sensor/RConn1 -- PS Lookup Table (1D)/LConn1
  PS Lookup Table (1D)/RConn1 -- Variable Resistor/LConn1

== system ssc_battery_management_R2020a/i_loads ==
  Current Sensor : fl_lib/Electrical/Electrical Sensors/Current Sensor
  PS-S : nesl_utility/PS-Simulink Converter  PhysicalDomain=network_engine_domain  SubClassName=ps_output  LeftPortType=input  RightPortType=output  PseudoPeriodic=off  Frequencies=[]  Unit=A  AffineConversion=off
  Terminator : Terminator
  current : Scope
  p : PMIOPort  Side=Left
  m : PMIOPort  Port=2  Side=Right
  wires:
  [i_loads] -> Terminator/1
  PS-S/1 -> [i_loads], current/1  "current"
  connections:
  Current Sensor/RConn1 -- PS-S/LConn1
  p/RConn1 -- Current Sensor/LConn1
  m/RConn1 -- Current Sensor/RConn2

== system ssc_battery_management_R2020a/power window ==
  PS Lookup Table (1D) : fl_lib/Physical Signals/Lookup Tables/PS Lookup Table (1D)  x=[0 voltage] V  f=[voltage(1)/current(1) voltage./current] Ohm  interp_method=simscape.enum.interpolation.linear  extrap_method=simscape.enum.extrapolation.nearest
      settings: SourceProductBaseCode=SS
  Variable Resistor : fl_lib/Electrical/Electrical Elements/Variable Resistor  Rmin=0.01 Ohm  i_specify=off  i_priority=None  i=0 A  i_nominal_specify=off  i_nominal_unit=A  i_nominal_value=1  v_specify=off  v_priority=None  v=0 V  v_nominal_specify=off  v_nominal_unit=V  v_nominal_value=1
  Voltage Sensor : fl_lib/Electrical/Electrical Sensors/Voltage Sensor
  + : PMIOPort  Tag=PMCPort  Side=Left
  - : PMIOPort  Tag=PMCPort  Port=2  Side=Right
  connections:
  Voltage Sensor/RConn2 -- Variable Resistor/RConn1 -- -/RConn1
  Voltage Sensor/LConn1 -- Variable Resistor/LConn2 -- +/RConn1
  Voltage Sensor/RConn1 -- PS Lookup Table (1D)/LConn1
  PS Lookup Table (1D)/RConn1 -- Variable Resistor/LConn1

== system ssc_battery_management_R2020a/radiator fan ==
  PS Lookup Table (1D) : fl_lib/Physical Signals/Lookup Tables/PS Lookup Table (1D)  x=[0 voltage] V  f=[voltage(1)/current(1) voltage./current] Ohm  interp_method=simscape.enum.interpolation.linear  extrap_method=simscape.enum.extrapolation.nearest
      settings: SourceProductBaseCode=SS
  Variable Resistor : fl_lib/Electrical/Electrical Elements/Variable Resistor  Rmin=0.01 Ohm  i_specify=off  i_priority=None  i=0 A  i_nominal_specify=off  i_nominal_unit=A  i_nominal_value=1  v_specify=off  v_priority=None  v=0 V  v_nominal_specify=off  v_nominal_unit=V  v_nominal_value=1
  Voltage Sensor : fl_lib/Electrical/Electrical Sensors/Voltage Sensor
  + : PMIOPort  Tag=PMCPort  Side=Left
  - : PMIOPort  Tag=PMCPort  Port=2  Side=Right
  connections:
  Voltage Sensor/RConn2 -- Variable Resistor/RConn1 -- -/RConn1
  Voltage Sensor/LConn1 -- Variable Resistor/LConn2 -- +/RConn1
  Voltage Sensor/RConn1 -- PS Lookup Table (1D)/LConn1
  PS Lookup Table (1D)/RConn1 -- Variable Resistor/LConn1

== system ssc_battery_management_R2020a/seat1 ==
  PS Lookup Table (1D) : fl_lib/Physical Signals/Lookup Tables/PS Lookup Table (1D)  x=[0 voltage] V  f=[voltage(1)/current(1) voltage./current] Ohm  interp_method=simscape.enum.interpolation.linear  extrap_method=simscape.enum.extrapolation.nearest
      settings: SourceProductBaseCode=SS
  Variable Resistor : fl_lib/Electrical/Electrical Elements/Variable Resistor  Rmin=0.01 Ohm  i_specify=off  i_priority=None  i=0 A  i_nominal_specify=off  i_nominal_unit=A  i_nominal_value=1  v_specify=off  v_priority=None  v=0 V  v_nominal_specify=off  v_nominal_unit=V  v_nominal_value=1
  Voltage Sensor : fl_lib/Electrical/Electrical Sensors/Voltage Sensor
  + : PMIOPort  Tag=PMCPort  Side=Left
  - : PMIOPort  Tag=PMCPort  Port=2  Side=Right
  connections:
  Voltage Sensor/RConn2 -- Variable Resistor/RConn1 -- -/RConn1
  Voltage Sensor/LConn1 -- Variable Resistor/LConn2 -- +/RConn1
  Voltage Sensor/RConn1 -- PS Lookup Table (1D)/LConn1
  PS Lookup Table (1D)/RConn1 -- Variable Resistor/LConn1
